simulink model "detectTrigger"  (R2016b)
settings: Solver=FixedStepDiscrete  StartTime=0.0  StopTime=Inf  FixedStep=sCoreParams.core.stepPeriod  RelTol=1e-3  EnableMultiTasking=on
undefined symbols (not defined in the file): sCoreParams
libraries: simulink x2, dspswit3 x2
settings Model: DataTypeOverride=Double  MinMaxOverflowLogging=ForceOff  Creator=rzelmann  LastModifiedBy=rzelmann
settings SolverCC: EnableConcurrentExecution=on
settings DataIOCC: SaveFormat=StructureWithTime
settings OptimizationCC: BlockReduction=off  DefaultParameterBehavior=Inlined  OptimizeBlockIOStorage=off  BufferReuse=off  GlobalBufferReuse=off  ExpressionFolding=off  LocalBlockOutputs=off  LifeSpan=inf
settings DebuggingCC: SFUnexpectedBacktrackingDiag=warning  SFNoUnconditionalDefaultTransitionDiag=warning  SFExecutionAtInitializationDiag=none
settings HardwareCC: ProdBitPerPointer=32  ProdBitPerSizeT=32  ProdBitPerPtrDiffT=32  ProdLargestAtomicFloat=None  ProdWordSize=32  ProdLongLongMode=on  ProdHWDeviceType=Generic->32-bit x86 compatible
settings ModelReferenceCC: ModelReferencePassRootInputsByReference=off
settings RTWCC: SystemTargetFile=slrt.tlc  TemplateMakefile=slrt_default_tmf  Description=Simulink Real-Time  RTWCompilerOptimization=on
settings ConfigComp: CovMetricSettings=dw  CovHtmlReporting=on  CovSaveCumulativeToWorkspaceVar=on  CovSaveSingleToWorkspaceVar=on  CovExternalEMLEnable=off

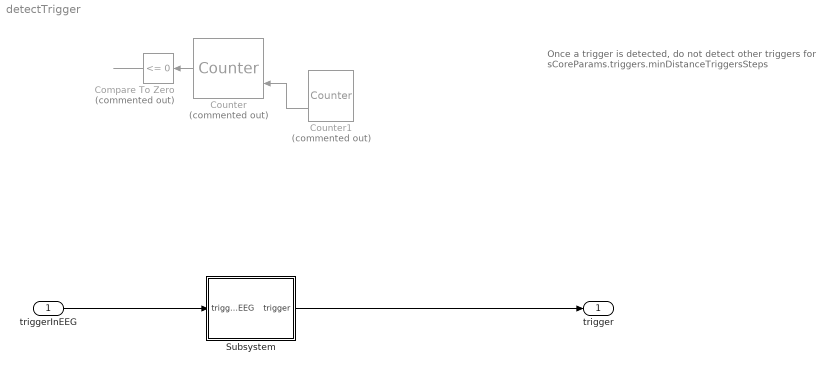
== system detectTrigger ==
  note: Once a trigger is detected,
      | do not detect other triggers for
      | sCoreParams.triggers.minDistanceTriggersSteps
  triggerInEEG : Inport  PortDimensions=[sCoreParams.core.samplesPerStep 1]
  Compare To Zero : simulink/Logic and Bit Operations/Compare To Zero  Commented=on  relop=<=  OutDataTypeStr=boolean
  Counter : dspswit3/Counter  Commented=on  Direction=Up  CountEvent=Rising edge  CounterSize=32 bits  MaxCount=255  InitialCount=0  Output=Count  HitValue=sCoreParams.triggers.minDistanceTriggersSamples  ResetInput=on  SamplesPerFrame=1  Ts=1  CntDtype=double  HitDtype=Logical
  Counter1 : dspswit3/Counter  Commented=on  Direction=Up  CountEvent=Free running  CounterSize=32 bits  MaxCount=255  InitialCount=0  Output=Count and Hit  HitValue=sCoreParams.triggers.minDistanceTriggersSteps  ResetInput=on  SamplesPerFrame=1  Ts=sCoreParams.core.stepPeriod  CntDtype=double  HitDtype=Logical
  Subsystem : Subsystem
  trigger : Outport
  wires:
  triggerInEEG/1 -> Subsystem/1(triggerInEEG)
  Subsystem/1(trigger) -> trigger/1
  ? -> Counter/1
  ? -> Counter1/1
  Counter/1 -> Compare To Zero/1
  Compare To Zero/1 -> ?
  Counter1/2 -> Counter/2

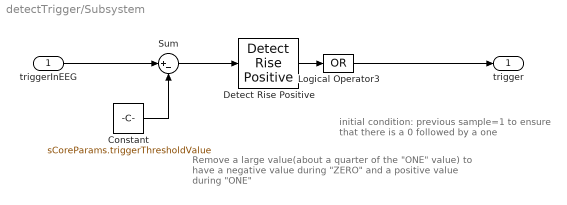
== system detectTrigger/Subsystem ==
  note: initial condition: previous sample=1 to ensure
      | that there is a 0 followed by a one
  note: Remove a large value(about a quarter of the "ONE" value)
      |  to have a negative value during "ZERO"
      | and a positive value during "ONE"
  triggerInEEG : Inport
  Constant : Constant  Value=sCoreParams.triggerThresholdValue
  Detect Rise Positive : simulink/Logic and Bit Operations/Detect Rise Positive  vinit=1  OutDataTypeStr=boolean
  Logical Operator3 : Logic  Operator=OR  Inputs=1  IconShape=distinctive  AllPortsSameDT=off  OutDataTypeStr=boolean
  Sum : Sum  Inputs=|+-
  trigger : Outport  OutputWhenDisabled=reset  InitialOutput=0
  wires:
  Constant/1 -> Sum/2
  Logical Operator3/1 -> trigger/1
  triggerInEEG/1 -> Sum/1
  Detect Rise Positive/1 -> Logical Operator3/1
  Sum/1 -> Detect Rise Positive/1
